simulink model "BLDC_Motor_FOC_rev3"  (R2017b)
settings: Solver=FixedStepDiscrete  StartTime=0.0  StopTime=2  MaxStep=1e-4  RelTol=1e-4
values from neighbouring files (symbols this model uses):
  A = 0    [control.m]
undefined symbols (not defined in the file or in its folder): DiscIntNeverNeededParam
libraries: powerlib x10, simulink x4
settings Model: Creator=Nick  LastModifiedBy=Nick
settings CodeAppCC: StateflowObjectComments=on

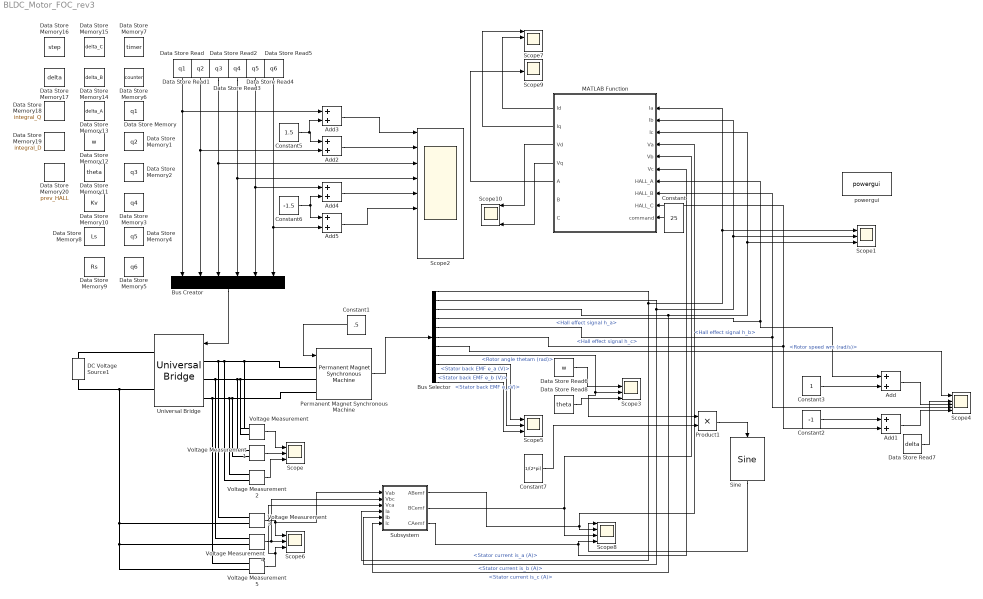
== system BLDC_Motor_FOC_rev3 ==
  Add{,1..5} (6 alike) : Sum
  Bus Creator : BusCreator  Inputs=6
  Bus Selector : BusSelector  OutputSignals=Stator current is_a (A),Stator current is_b (A),Stator current is_c (A),Hall effect signal h_a,Hall effect signal h_b,Hall effect signal h_c,Rotor speed wm (rad/s),Rotor angle thetam (rad),Stator back EMF e_a (V),Stator back EMF e_b (V),Stator back EMF e_cV)
  Constant : Constant  Value=25
  Constant1 : Constant  Value=.5
  Constant2 : Constant  Value=-1
  Constant3 : Constant
  Constant5 : Constant  Value=1.5
  Constant6 : Constant  Value=-1.5
  Constant7 : Constant  Value=1/(2*pi)
  DC Voltage Source1 : powerlib/Electrical Sources/DC Voltage Source  Amplitude=48  Measurements=None
  Data Store Memory : DataStoreMemory  DataStoreName=q1  ReadBeforeWriteMsg=warning  WriteAfterWriteMsg=warning  WriteAfterReadMsg=warning  ShowAdditionalParam=off  OutDataTypeStr=double
  Data Store Memory1 : DataStoreMemory  DataStoreName=q2  ReadBeforeWriteMsg=warning  WriteAfterWriteMsg=warning  WriteAfterReadMsg=warning  ShowAdditionalParam=off  OutDataTypeStr=double
  Data Store Memory10 : DataStoreMemory  DataStoreName=Kv  ReadBeforeWriteMsg=warning  WriteAfterWriteMsg=warning  WriteAfterReadMsg=warning  InitialValue=100  ShowAdditionalParam=off  OutDataTypeStr=double
  Data Store Memory11 : DataStoreMemory  DataStoreName=theta  ReadBeforeWriteMsg=warning  WriteAfterWriteMsg=warning  WriteAfterReadMsg=warning  ShowAdditionalParam=off  OutDataTypeStr=double
  Data Store Memory12 : DataStoreMemory  DataStoreName=w  ReadBeforeWriteMsg=warning  WriteAfterWriteMsg=warning  WriteAfterReadMsg=warning  ShowAdditionalParam=off  OutDataTypeStr=double
  Data Store Memory13 : DataStoreMemory  DataStoreName=delta_A  ReadBeforeWriteMsg=warning  WriteAfterWriteMsg=warning  WriteAfterReadMsg=warning  ShowAdditionalParam=off  OutDataTypeStr=double
  Data Store Memory14 : DataStoreMemory  DataStoreName=delta_B  ReadBeforeWriteMsg=warning  WriteAfterWriteMsg=warning  WriteAfterReadMsg=warning  ShowAdditionalParam=off  OutDataTypeStr=double
  Data Store Memory15 : DataStoreMemory  DataStoreName=delta_C  ReadBeforeWriteMsg=warning  WriteAfterWriteMsg=warning  WriteAfterReadMsg=warning  ShowAdditionalParam=off  OutDataTypeStr=double
  Data Store Memory16 : DataStoreMemory  DataStoreName=step  ReadBeforeWriteMsg=warning  WriteAfterWriteMsg=warning  WriteAfterReadMsg=warning  InitialValue=5e-6  ShowAdditionalParam=off  OutDataTypeStr=double
  Data Store Memory17 : DataStoreMemory  DataStoreName=delta  ReadBeforeWriteMsg=warning  WriteAfterWriteMsg=warning  WriteAfterReadMsg=warning  ShowAdditionalParam=off  OutDataTypeStr=double
  Data Store Memory18 : DataStoreMemory  DataStoreName=integral_Q  ReadBeforeWriteMsg=warning  WriteAfterWriteMsg=warning  WriteAfterReadMsg=warning  ShowAdditionalParam=off  OutDataTypeStr=double
  Data Store Memory19 : DataStoreMemory  DataStoreName=integral_D  ReadBeforeWriteMsg=warning  WriteAfterWriteMsg=warning  WriteAfterReadMsg=warning  ShowAdditionalParam=off  OutDataTypeStr=double
  Data Store Memory2 : DataStoreMemory  DataStoreName=q3  ReadBeforeWriteMsg=warning  WriteAfterWriteMsg=warning  WriteAfterReadMsg=warning  ShowAdditionalParam=off  OutDataTypeStr=double
  Data Store Memory20 : DataStoreMemory  DataStoreName=prev_HALL  ReadBeforeWriteMsg=warning  WriteAfterWriteMsg=warning  WriteAfterReadMsg=warning  ShowAdditionalParam=off  OutDataTypeStr=double
  Data Store Memory3 : DataStoreMemory  DataStoreName=q4  ReadBeforeWriteMsg=warning  WriteAfterWriteMsg=warning  WriteAfterReadMsg=warning  ShowAdditionalParam=off  OutDataTypeStr=double
  Data Store Memory4 : DataStoreMemory  DataStoreName=q5  ReadBeforeWriteMsg=warning  WriteAfterWriteMsg=warning  WriteAfterReadMsg=warning  ShowAdditionalParam=off  OutDataTypeStr=double
  Data Store Memory5 : DataStoreMemory  DataStoreName=q6  ReadBeforeWriteMsg=warning  WriteAfterWriteMsg=warning  WriteAfterReadMsg=warning  ShowAdditionalParam=off  OutDataTypeStr=double
  Data Store Memory6 : DataStoreMemory  DataStoreName=counter  ReadBeforeWriteMsg=warning  WriteAfterWriteMsg=warning  WriteAfterReadMsg=warning  ShowAdditionalParam=off  OutDataTypeStr=double
  Data Store Memory7 : DataStoreMemory  DataStoreName=timer  ReadBeforeWriteMsg=warning  WriteAfterWriteMsg=warning  WriteAfterReadMsg=warning  ShowAdditionalParam=off  OutDataTypeStr=double
  Data Store Memory8 : DataStoreMemory  DataStoreName=Ls  ReadBeforeWriteMsg=warning  WriteAfterWriteMsg=warning  WriteAfterReadMsg=warning  InitialValue=.0085  ShowAdditionalParam=off  OutDataTypeStr=double
  Data Store Memory9 : DataStoreMemory  DataStoreName=Rs  ReadBeforeWriteMsg=warning  WriteAfterWriteMsg=warning  WriteAfterReadMsg=warning  InitialValue=.0485  ShowAdditionalParam=off  OutDataTypeStr=double
  Data Store Read : DataStoreRead  DataStoreName=q1
  Data Store Read1 : DataStoreRead  DataStoreName=q2
  Data Store Read2 : DataStoreRead  DataStoreName=q3
  Data Store Read3 : DataStoreRead  DataStoreName=q4
  Data Store Read4 : DataStoreRead  DataStoreName=q5
  Data Store Read5 : DataStoreRead  DataStoreName=q6
  Data Store Read6 : DataStoreRead  DataStoreName=w
  Data Store Read7 : DataStoreRead  DataStoreName=delta
  Data Store Read8 : DataStoreRead  DataStoreName=theta
  MATLAB Function : MATLAB Function  TreatAsAtomicUnit=on
  Permanent Magnet Synchronous Machine : powerlib/Machines/Permanent Magnet Synchronous Machine  NbPhases=3  FluxDistribution=Trapezoidal  RotorType=Round  MechanicalLoad=Torque Tm  PresetModel=No  ShowDetailedParameters=on  MeasurementBus=off  Resistance=0.0485  Inductance=8.5e-3  dqInductances=[8.5e-3,8.5e-3]  La=0.000395  MachineConstant=Flux linkage established by magnets (V.s)  Flux=0.1194  VoltageCst=100.0283  TorqueCst=0.9552  Flat=120  Mechanical=[0.0027 0.0004924 4 0]  PolePairs=4  InitialConditions=[0,0, 0,0]  InitialConditions5ph=[0 0 0 0 0 0]  TsPowergui=0  TsBlock=-1  RefAngle=90 degrees behind phase A axis (modified Park)
      settings: SourceProductName=Simscape Power Systems
  Product1 : Product
  Scope{,1,5..6} (4 alike) : Scope  NumInputPorts=3
  Scope{3,7..8,10} (4 alike) : Scope  NumInputPorts=4
  Scope2 : Scope  NumInputPorts=9
  Scope4 : Scope  NumInputPorts=6
  Scope9 : Scope  NumInputPorts=6
  Sine : simulink/Lookup Tables/Sine  Formula=sin(2*pi*u)  NumDataPoints=(2^5)+1  OutputWordLength=16  InternalRulePriority=Speed
      settings: SourceProductName=Simulink
  Subsystem : Subsystem
  Universal Bridge : powerlib/Power Electronics/Universal Bridge  Arms=3  SnubberResistance=1e5  SnubberCapacitance=inf  Device=MOSFET / Diodes  Ron=1e-3  Lon=0  ForwardVoltages="[  0  0  ]"  ForwardVoltage=0  GTOparameters=[ 10e-6 , 20e-6 ]  IGBTparameters=[ 1e-6 , 2e-6 ]  Measurements=None  Measurements_2=None  converterType=Rectifier
  Voltage Measurement{,1..5} (6 alike) : powerlib/Measurements/Voltage Measurement  PhasorSimulation=off  OutputType=Complex  PSBequivalent=0
  powergui : powerlib/powergui  Priority=1  SimulationMode=Discrete  SampleTime=5e-5  frequency=60  Iterations=50  frequencyindice=0  Pbase=100e6  ErrMax=1e-4  UnitsV=kV  UnitsW=MW  buscounter=0  FunctionMessages=off  echomessages=off  EnableUseOfTLC=off  CurrentSourceSwitches=off  DisableSnubberDevices=off  DisableRonSwitches=off  DisableVfSwitches=off  DisplayEquations=off  SolverType=Tustin/Backward Euler (TBE)  Interpol=off  ExternalGateDelay=off  methode=off  Ts=100  x0status=blocks  SPID=off  SwTol=0  HookPort=off  RestoreLinks=warning  ResistiveCurrentMeasurement=off  Frange=[0:2:500]  Ylog=off  Xlog=on  ShowGrid=off  save=off  variable=ZData  structure=0  ZoomFFT=off  StartTime=0.0  cycles=1  DisplayStyle=1  fundamental=60  FreqAxis=off  MaxFrequency=1000  frequencyindicesteady=1  RmsSteady=1  display=off
  wires:
  Permanent Magnet Synchronous Machine/1 -> Bus Selector/1
  Bus Selector/1 -> Subsystem/4(Ia), MATLAB Function/1(Ia), Scope1/1  "<Stator current is_a (A)>"
  Constant/1 -> MATLAB Function/10(command)
  Bus Selector/5 -> Scope4/5, MATLAB Function/8(HALL_B)  "<Hall effect signal h_b>"
  Bus Selector/6 -> Add1/2, MATLAB Function/9(HALL_C)  "<Hall effect signal h_c>"
  Bus Selector/4 -> Add/1, MATLAB Function/7(HALL_A)  "<Hall effect signal h_a>"
  Voltage Measurement/1 -> Scope/1
  Bus Creator/1 -> Universal Bridge/1
  Constant3/1 -> Add/2
  Constant2/1 -> Add1/1
  Add1/1 -> Scope4/6
  Add/1 -> Scope4/4
  Data Store Read/1 -> Add3/1, Bus Creator/1
  Data Store Read2/1 -> Scope2/3, Bus Creator/3
  Data Store Read3/1 -> Scope2/4, Bus Creator/4
  Data Store Read4/1 -> Add4/1, Bus Creator/5
  Constant1/1 -> Permanent Magnet Synchronous Machine/1
  Bus Selector/7 -> Scope4/1  "<Rotor speed wm (rad/s)>"
  Voltage Measurement4/1 -> Subsystem/2(Vbc), Scope6/2
  Voltage Measurement5/1 -> Subsystem/3(Vca), Scope6/3
  Data Store Read1/1 -> Add2/2, Bus Creator/2
  Bus Selector/8 -> Scope3/3, Product1/1  "<Rotor angle thetam (rad)>"
  Add2/1 -> Scope2/2
  Constant5/1 -> Add3/2, Add2/1
  Add4/1 -> Scope2/5
  Add5/1 -> Scope2/6
  Constant6/1 -> Add5/1, Add4/2
  Data Store Read5/1 -> Add5/2, Bus Creator/6
  Bus Selector/9 -> Scope5/1  "<Stator back EMF e_a (V)>"
  Bus Selector/10 -> Scope5/2  "<Stator back EMF e_b (V)>"
  Bus Selector/11 -> Scope5/3  "<Stator back EMF e_cV)>"
  Add3/1 -> Scope2/1
  Voltage Measurement3/1 -> Subsystem/1(Vab), Scope6/1
  Bus Selector/2 -> Subsystem/5(Ib), MATLAB Function/2(Ib), Scope1/2  "<Stator current is_b (A)>"
  Bus Selector/3 -> Subsystem/6(Ic), MATLAB Function/3(Ic), Scope1/3  "<Stator current is_c (A)>"
  Voltage Measurement1/1 -> Scope/2
  Voltage Measurement2/1 -> Scope/3
  Constant7/1 -> Product1/2
  Product1/1 -> Sine/1
  Sine/1 -> Scope8/1
  Subsystem/1(ABemf) -> MATLAB Function/4(Va), Scope8/2
  Subsystem/2(BCemf) -> MATLAB Function/5(Vb), Scope8/3
  Subsystem/3(CAemf) -> MATLAB Function/6(Vc), Scope8/4
  Data Store Read6/1 -> Scope3/2
  Data Store Read7/1 -> Scope4/3
  MATLAB Function/1(Id) -> Scope7/2
  MATLAB Function/2(Iq) -> Scope7/1
  Data Store Read8/1 -> Scope3/4
  MATLAB Function/3(Vd) -> Scope10/1
  MATLAB Function/4(Vq) -> Scope10/4
  MATLAB Function/5(A) -> Scope9/4
  connections:
  Universal Bridge/LConn1 -- Voltage Measurement3/LConn1 -- Voltage Measurement2/LConn2 -- Voltage Measurement/LConn1 -- Permanent Magnet Synchronous Machine/LConn1
  Universal Bridge/LConn2 -- Voltage Measurement4/LConn1 -- Voltage Measurement1/LConn1 -- Permanent Magnet Synchronous Machine/LConn2 -- Voltage Measurement/LConn2
  Universal Bridge/LConn3 -- Voltage Measurement5/LConn1 -- Voltage Measurement2/LConn1 -- Permanent Magnet Synchronous Machine/LConn3 -- Voltage Measurement1/LConn2
  Universal Bridge/RConn1 -- DC Voltage Source1/RConn1
  Universal Bridge/RConn2 -- Voltage Measurement3/LConn2 -- Voltage Measurement4/LConn2 -- Voltage Measurement5/LConn2 -- DC Voltage Source1/LConn1

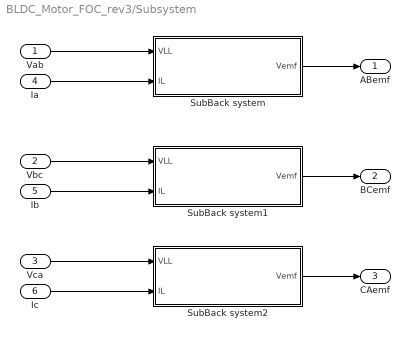
== system BLDC_Motor_FOC_rev3/Subsystem ==
  Vab : Inport
  Vbc : Inport  Port=2
  Vca : Inport  Port=3
  Ia : Inport  Port=4
  Ib : Inport  Port=5
  Ic : Inport  Port=6
  SubBack system : Subsystem  mask{Parameter1=on}
  SubBack system1 : Subsystem  mask{Parameter1=on}
  SubBack system2 : Subsystem  mask{Parameter1=on}
  ABemf : Outport
  BCemf : Outport  Port=2
  CAemf : Outport  Port=3
  wires:
  Vab/1 -> SubBack system/1(VLL)
  Ia/1 -> SubBack system/2(IL)
  SubBack system/1(Vemf) -> ABemf/1
  Vbc/1 -> SubBack system1/1(VLL)
  Ib/1 -> SubBack system1/2(IL)
  SubBack system1/1(Vemf) -> BCemf/1
  Vca/1 -> SubBack system2/1(VLL)
  Ic/1 -> SubBack system2/2(IL)
  SubBack system2/1(Vemf) -> CAemf/1

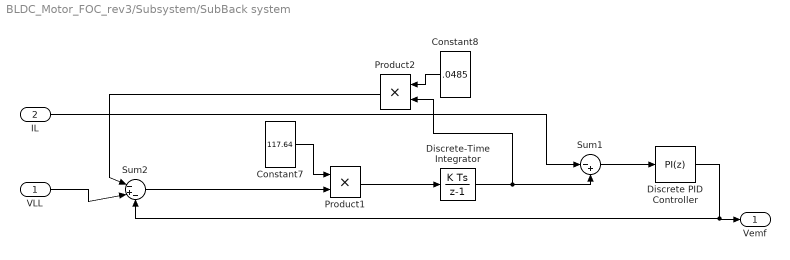
== system BLDC_Motor_FOC_rev3/Subsystem/SubBack system ==
  VLL : Inport
  IL : Inport  Port=2
  Constant7 : Constant  Value=117.64
  Constant8 : Constant  Value=.0485
  Discrete PID Controller : simulink/Continuous/PID Controller  Controller=PI  TimeDomain=Discrete-time  SampleTime=-1  IntegratorMethod=Forward Euler  FilterMethod=Forward Euler  Form=Parallel  UseFilter=on  ControllerParametersSource=internal  P=1  I=5  D=0  N=100  InitialConditionSource=internal  InitialConditionForIntegrator=0  InitialConditionForFilter=0  ExternalReset=none  LimitOutput=off  UpperSaturationLimit=inf  LowerSaturationLimit=-inf  LinearizeAsGain=off  AntiWindupMode=none  Kb=1  TrackingMode=off  Kt=1  PParamMin=[]  PParamMax=[]  IParamMin=[]  IParamMax=[]  DParamMin=[]  DParamMax=[]  NParamMin=[]  NParamMax=[]  KbParamMin=[]  KbParamMax=[]  KtParamMin=[]  KtParamMax=[]  POutMin=[]  POutMax=[]  IOutMin=[]  IOutMax=[]  DOutMin=[]  DOutMax=[]  NOutMin=[]  NOutMax=[]  KbOutMin=[]  KbOutMax=[]  KtOutMin=[]  KtOutMax=[]  IntegratorOutMin=[]  IntegratorOutMax=[]  FilterOutMin=[]  FilterOutMax=[]  SumOutMin=[]  SumOutMax=[]  SumI1OutMin=[]  SumI1OutMax=[]  SumI2OutMin=[]  SumI2OutMax=[]  SumI3OutMin=[]  SumI3OutMax=[]  SumDOutMin=[]  SumDOutMax=[]  SaturationOutMin=[]  SaturationOutMax=[]  IntegratorContinuousStateAttributes=''  IntegratorStateMustResolveToSignalObject=off  IntegratorRTWStateStorageClass=Auto  FilterContinuousStateAttributes=''  FilterStateMustResolveToSignalObject=off  FilterRTWStateStorageClass=Auto  DifferentiatorICPrevScaledInput=0  DifferentiatorOutMin=[]  DifferentiatorOutMax=[]  InitialConditionSetting=State (most efficient)  FilterDiffOutCoefMin=[]  FilterDiffOutCoefMax=[]  SumDenOutMin=[]  SumDenOutMax=[]  SumNumOutMin=[]  SumNumOutMax=[]  ReciprocalOutMin=[]  ReciprocalOutMax=[]  DivideOutMin=[]  DivideOutMax=[]  TunerSelectOption=Transfer Function Based (PID Tuner App)
  Discrete-Time Integrator : DiscreteIntegrator  InitialConditionSetting=State (most efficient)  SampleTime=-1  ICPrevOutput=DiscIntNeverNeededParam  ICPrevScaledInput=DiscIntNeverNeededParam
  Product1 : Product
  Product2 : Product
  Sum1 : Sum  Inputs=|-+
  Sum2 : Sum  Inputs=|-+-
  Vemf : Outport
  wires:
  IL/1 -> Sum1/1
  Sum1/1 -> Discrete PID Controller/1
  Discrete-Time Integrator/1 -> Product2/2, Sum1/2
  VLL/1 -> Sum2/2
  Sum2/1 -> Product1/2
  Constant7/1 -> Product1/1
  Product2/1 -> Sum2/1
  Constant8/1 -> Product2/1
  Discrete PID Controller/1 -> Vemf/1, Sum2/3
  Product1/1 -> Discrete-Time Integrator/1

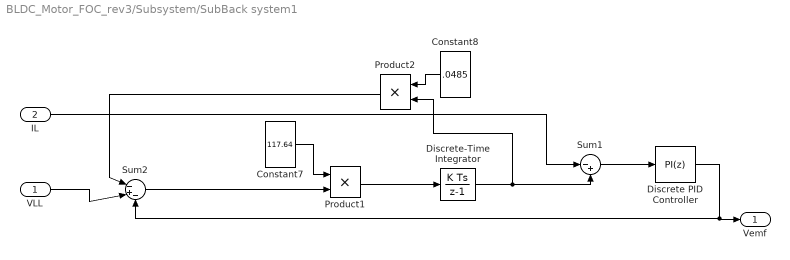
== system BLDC_Motor_FOC_rev3/Subsystem/SubBack system1 ==
  VLL : Inport
  IL : Inport  Port=2
  Constant7 : Constant  Value=117.64
  Constant8 : Constant  Value=.0485
  Discrete PID Controller : simulink/Continuous/PID Controller  Controller=PI  TimeDomain=Discrete-time  SampleTime=-1  IntegratorMethod=Forward Euler  FilterMethod=Forward Euler  Form=Parallel  UseFilter=on  ControllerParametersSource=internal  P=1  I=5  D=0  N=100  InitialConditionSource=internal  InitialConditionForIntegrator=0  InitialConditionForFilter=0  ExternalReset=none  LimitOutput=off  UpperSaturationLimit=inf  LowerSaturationLimit=-inf  LinearizeAsGain=off  AntiWindupMode=none  Kb=1  TrackingMode=off  Kt=1  PParamMin=[]  PParamMax=[]  IParamMin=[]  IParamMax=[]  DParamMin=[]  DParamMax=[]  NParamMin=[]  NParamMax=[]  KbParamMin=[]  KbParamMax=[]  KtParamMin=[]  KtParamMax=[]  POutMin=[]  POutMax=[]  IOutMin=[]  IOutMax=[]  DOutMin=[]  DOutMax=[]  NOutMin=[]  NOutMax=[]  KbOutMin=[]  KbOutMax=[]  KtOutMin=[]  KtOutMax=[]  IntegratorOutMin=[]  IntegratorOutMax=[]  FilterOutMin=[]  FilterOutMax=[]  SumOutMin=[]  SumOutMax=[]  SumI1OutMin=[]  SumI1OutMax=[]  SumI2OutMin=[]  SumI2OutMax=[]  SumI3OutMin=[]  SumI3OutMax=[]  SumDOutMin=[]  SumDOutMax=[]  SaturationOutMin=[]  SaturationOutMax=[]  IntegratorContinuousStateAttributes=''  IntegratorStateMustResolveToSignalObject=off  IntegratorRTWStateStorageClass=Auto  FilterContinuousStateAttributes=''  FilterStateMustResolveToSignalObject=off  FilterRTWStateStorageClass=Auto  DifferentiatorICPrevScaledInput=0  DifferentiatorOutMin=[]  DifferentiatorOutMax=[]  InitialConditionSetting=State (most efficient)  FilterDiffOutCoefMin=[]  FilterDiffOutCoefMax=[]  SumDenOutMin=[]  SumDenOutMax=[]  SumNumOutMin=[]  SumNumOutMax=[]  ReciprocalOutMin=[]  ReciprocalOutMax=[]  DivideOutMin=[]  DivideOutMax=[]  TunerSelectOption=Transfer Function Based (PID Tuner App)
  Discrete-Time Integrator : DiscreteIntegrator  InitialConditionSetting=State (most efficient)  SampleTime=-1  ICPrevOutput=DiscIntNeverNeededParam  ICPrevScaledInput=DiscIntNeverNeededParam
  Product1 : Product
  Product2 : Product
  Sum1 : Sum  Inputs=|-+
  Sum2 : Sum  Inputs=|-+-
  Vemf : Outport
  wires:
  Product1/1 -> Discrete-Time Integrator/1
  Discrete PID Controller/1 -> Sum2/3, Vemf/1
  Constant8/1 -> Product2/1
  Product2/1 -> Sum2/1
  Constant7/1 -> Product1/1
  Sum2/1 -> Product1/2
  VLL/1 -> Sum2/2
  Discrete-Time Integrator/1 -> Sum1/2, Product2/2
  Sum1/1 -> Discrete PID Controller/1
  IL/1 -> Sum1/1

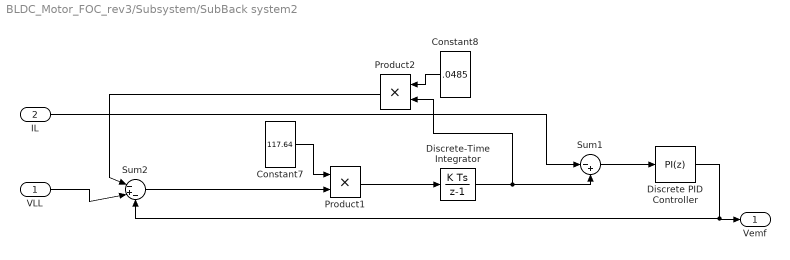
== system BLDC_Motor_FOC_rev3/Subsystem/SubBack system2 ==
  VLL : Inport
  IL : Inport  Port=2
  Constant7 : Constant  Value=117.64
  Constant8 : Constant  Value=.0485
  Discrete PID Controller : simulink/Continuous/PID Controller  Controller=PI  TimeDomain=Discrete-time  SampleTime=-1  IntegratorMethod=Forward Euler  FilterMethod=Forward Euler  Form=Parallel  UseFilter=on  ControllerParametersSource=internal  P=1  I=5  D=0  N=100  InitialConditionSource=internal  InitialConditionForIntegrator=0  InitialConditionForFilter=0  ExternalReset=none  LimitOutput=off  UpperSaturationLimit=inf  LowerSaturationLimit=-inf  LinearizeAsGain=off  AntiWindupMode=none  Kb=1  TrackingMode=off  Kt=1  PParamMin=[]  PParamMax=[]  IParamMin=[]  IParamMax=[]  DParamMin=[]  DParamMax=[]  NParamMin=[]  NParamMax=[]  KbParamMin=[]  KbParamMax=[]  KtParamMin=[]  KtParamMax=[]  POutMin=[]  POutMax=[]  IOutMin=[]  IOutMax=[]  DOutMin=[]  DOutMax=[]  NOutMin=[]  NOutMax=[]  KbOutMin=[]  KbOutMax=[]  KtOutMin=[]  KtOutMax=[]  IntegratorOutMin=[]  IntegratorOutMax=[]  FilterOutMin=[]  FilterOutMax=[]  SumOutMin=[]  SumOutMax=[]  SumI1OutMin=[]  SumI1OutMax=[]  SumI2OutMin=[]  SumI2OutMax=[]  SumI3OutMin=[]  SumI3OutMax=[]  SumDOutMin=[]  SumDOutMax=[]  SaturationOutMin=[]  SaturationOutMax=[]  IntegratorContinuousStateAttributes=''  IntegratorStateMustResolveToSignalObject=off  IntegratorRTWStateStorageClass=Auto  FilterContinuousStateAttributes=''  FilterStateMustResolveToSignalObject=off  FilterRTWStateStorageClass=Auto  DifferentiatorICPrevScaledInput=0  DifferentiatorOutMin=[]  DifferentiatorOutMax=[]  InitialConditionSetting=State (most efficient)  FilterDiffOutCoefMin=[]  FilterDiffOutCoefMax=[]  SumDenOutMin=[]  SumDenOutMax=[]  SumNumOutMin=[]  SumNumOutMax=[]  ReciprocalOutMin=[]  ReciprocalOutMax=[]  DivideOutMin=[]  DivideOutMax=[]  TunerSelectOption=Transfer Function Based (PID Tuner App)
  Discrete-Time Integrator : DiscreteIntegrator  InitialConditionSetting=State (most efficient)  SampleTime=-1  ICPrevOutput=DiscIntNeverNeededParam  ICPrevScaledInput=DiscIntNeverNeededParam
  Product1 : Product
  Product2 : Product
  Sum1 : Sum  Inputs=|-+
  Sum2 : Sum  Inputs=|-+-
  Vemf : Outport
  wires:
  IL/1 -> Sum1/1
  Sum1/1 -> Discrete PID Controller/1
  Discrete-Time Integrator/1 -> Product2/2, Sum1/2
  VLL/1 -> Sum2/2
  Sum2/1 -> Product1/2
  Constant7/1 -> Product1/1
  Product2/1 -> Sum2/1
  Constant8/1 -> Product2/1
  Discrete PID Controller/1 -> Vemf/1, Sum2/3
  Product1/1 -> Discrete-Time Integrator/1

== matlab function BLDC_Motor_FOC_rev3/MATLAB Function ==
  settings: updateMethod=DISCRETE  sampleTime=50e-7
  data: Id output; Iq output; Vd output; Vq output; Ia input size=1; Ib input size=1; Ic input size=1; Va input; Vb input; Vc input; HALL_A input; HALL_B input; HALL_C input size=1; command input size=1; q1 data_store_memory; q2 data_store_memory; q3 data_store_memory; q4 data_store_memory; q5 data_store_memory; q6 data_store_memory; counter data_store_memory; timer data_store_memory; A output; B output; C output; theta data_store_memory; Kv data_store_memory; w data_store_memory; delta_A data_store_memory; delta_B data_store_memory; delta_C data_store_memory; step data_store_memory; delta data_store_memory; integral_Q data_store_memory; integral_D data_store_memory; prev_HALL data_store_memory
function [Id,Iq,Vd,Vq,A,B,C] = control(Ia,Ib,Ic,Va,Vb,Vc,HALL_A,HALL_B,HALL_C,command)
global q1 
global q2 
global q3 
global q4 
global q5 
global q6
global counter
global delta
global step
global delta_A
global delta_B
global delta_C
global w
global theta
global timer
global integral_Q
global integral_D
global prev_HALL

A = 0;
B = 0;
C = 0;


[I_alpha,I_beta] = clarke(Ia,Ib,Ic);
[V_alpha,V_beta] = clarke(Va,Vb,Vc);

delta = delta + step;
timer = timer + step;

if((HALL_A-delta_A ~= 0 || HALL_B-delta_B ~= 0 || HALL_C-delta_C ~= 0))
    
    if HALL_A-delta_A == -1
        if prev_HALL == 3
            w = -1*((2*pi)/24)/delta;
            
        elseif prev_HALL == 2
            w = ((2*pi)/24)/delta;
        else
            w = 0;
            
        end
        prev_HALL = 1;
    
    elseif HALL_A-delta_A == 1
        if prev_HALL == 3
            w = -1*((2*pi)/24)/delta;
            
        elseif prev_HALL == 2
            w = ((2*pi)/24)/delta;
        else
            w = 0;
           
        end
        prev_HALL = 1;
    
    elseif HALL_B-delta_B == -1
        if prev_HALL == 1
            w = -1*((2*pi)/24)/delta;
            
        elseif prev_HALL == 3
            w = ((2*pi)/24)/delta;
            
        else
            w = 0;
            
        end
        prev_HALL = 2;
    
    elseif HALL_B-delta_B == 1
        if prev_HALL == 1
            w = -1*((2*pi)/24)/delta;
          
        elseif prev_HALL == 3
            w = ((2*pi)/24)/delta;
            
        else
            w = 0;
           
        end
        prev_HALL = 2;
    
    elseif HALL_C-delta_C == -1
        if prev_HALL == 2
            w = -1*((2*pi)/24)/delta;
            
        elseif prev_HALL == 1
            w = ((2*pi)/24)/delta;
            
        else
            w = 0;
            
        end
        prev_HALL = 3;

    elseif HALL_C-delta_C == 1
        if prev_HALL == 1
            w = ((2*pi)/24)/delta;
            
        elseif prev_HALL == 2
            w = -1*((2*pi)/24)/delta;
            
        else
            w = 0;
            
        end
        prev_HALL = 3;

    end
    
    delta = 0;
end


delta_A = HALL_A;
delta_B = HALL_B;
delta_C = HALL_C;
if timer > .03
    
    theta = theta + w*step;
end

[Id,Iq] = parke(I_alpha,I_beta,4*theta);
[Vd,Vq] = parke(V_alpha,V_beta,4*theta);





counter = counter + 1;
if timer < .1
    if counter <= command
        if HALL_A && ~HALL_B && HALL_C
            q1 = 1;
            q2 = 0;
            q3 = 0;
            q4 = 1;
            q5 = 1;
            q6 = 0;

        elseif HALL_A && ~HALL_B && ~HALL_C
            q1 = 1;
            q2 = 0;
            q3 = 0;
            q4 = 1;
            q5 = 0;
            q6 = 1;

        elseif HALL_A && HALL_B && ~HALL_C
            q1 = 1;
            q2 = 0;
            q3 = 1;
            q4 = 0;
            q5 = 0;
            q6 = 1;

        elseif ~HALL_A && HALL_B && ~HALL_C
            q1 = 0;
            q2 = 1;
            q3 = 1;
            q4 = 0;
            q5 = 0;
            q6 = 1;

        elseif ~HALL_A && HALL_B && HALL_C
            q1 = 0;
            q2 = 1;
            q3 = 1;
            q4 = 0;
            q5 = 1;
            q6 = 0; 

        elseif ~HALL_A && ~HALL_B && HALL_C
            q1 = 0;
            q2 = 1;
            q3 = 0;
            q4 = 1;
            q5 = 1;
            q6 = 0;
        end
    else
        q1 = 0;
        q2 = 0;
        q3 = 0;
        q4 = 0;
        q5 = 0;
        q6 = 0;
    end
    if counter >= 100
        counter = 0;
    end

else
    error_Q = (-(command/100)*30) - Iq;
    integral_Q = integral_Q + (error_Q*step);
    proportion_Q = error_Q;
    u_Q = 400*integral_Q + 400*proportion_Q;
    
    error_D = (0 - Id);
    integral_D = integral_D + (error_D*step);
    proportion_D = error_D;
    u_D = 400*integral_Q + 450*proportion_D;
    
    
    [I_alpha,I_beta] = inverse_parke(u_D,u_Q,4*theta);
    
    [A,B,C] = inverse_clarke(I_alpha,I_beta);
    regulate(A,B,C,Va,Vb,Vc);
end
    
end


function regulate(command_A,command_B,command_C,Va,Vb,Vc)
    global counter
    global q1
    global q2
    global q3
    global q4
    global q5
    global q6
    
    if Va < command_A
        q1 = 1;
        q2 = 0;
    else
        q1 = 0;
        q2 = 1;
    end
    if Vb < command_B
        q3 = 1;
        q4 = 0;
    else
        q3 = 0;
        q4 = 1;
    end
    if Vc < command_C
        q5 = 1;
        q6 = 0;
    else
        q5 = 0;
        q6 = 1;
    end

    counter = counter + 1;
    if counter >= 100
        counter = 0;
    end

end

function [d,q] = parke(alpha,beta,theta)
    d = cos(theta)*alpha + sin(theta)*beta;
    q = cos(theta)*beta - sin(theta)*alpha;
end

function [alpha,beta] = clarke(a,b,c)
    alpha = a;
    beta = (1/(sqrt(3))*(b-c));
end

function [alpha,beta] = inverse_parke(d,q,theta)
    alpha = d*cos(theta) - q*sin(theta);
    beta = q*cos(theta) + d*sin(theta);
end

function [a,b,c] = inverse_clarke(alpha,beta)
    a = alpha;
    b = (1/2)*((-alpha) + (sqrt(3)*beta));
    c = (1/2)*((-alpha) - (sqrt(3)*beta));
end
